simulink model "untitled1"  (R2025a)
settings: Solver=VariableStepAuto  StartTime=0.0  StopTime=36  MaxStep=1e-4  RelTol=1e-3
values from neighbouring files (symbols this model uses):
  alpha = 50    [Planning_Adaptive_LTV.m]
  beta = 5    [Planning_Adaptive_LTV.m]
  gamma = 10    [Planning_Adaptive_LTV.m]
  initial_positions_rad = rawJointPositions(1, :)'    [manipulator_sim.m]
  N = numel(theta_points_rad)    [create_LPV_linearizer.m]
  waypoints = pathObj.States(:, 1:2)    [Planning_Adaptive_LTV.m]
  x0 = zeros(10, 1)    [Planning_Adaptive_LTV.m]
undefined symbols (not defined in the file or in its folder): p, X, Y, Z
libraries: sm_lib x181, nesl_utility x29, fl_lib x3, simulink x2, eeGeneralControl x1
(part 1 of 5)
settings Model: Creator=chiar_zjcy1by  LastModifiedBy=chiar_zjcy1by

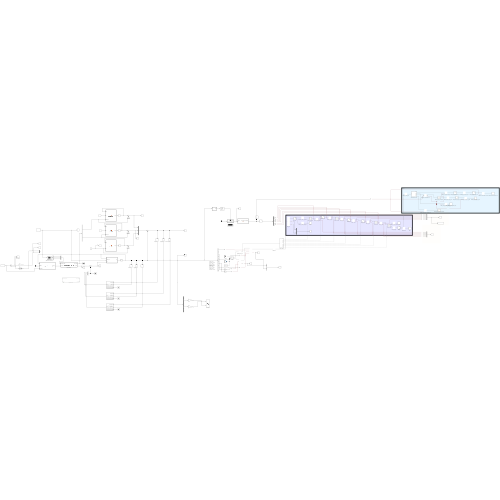
[thumbnail: Simulink's stored preview of the top-level diagram]
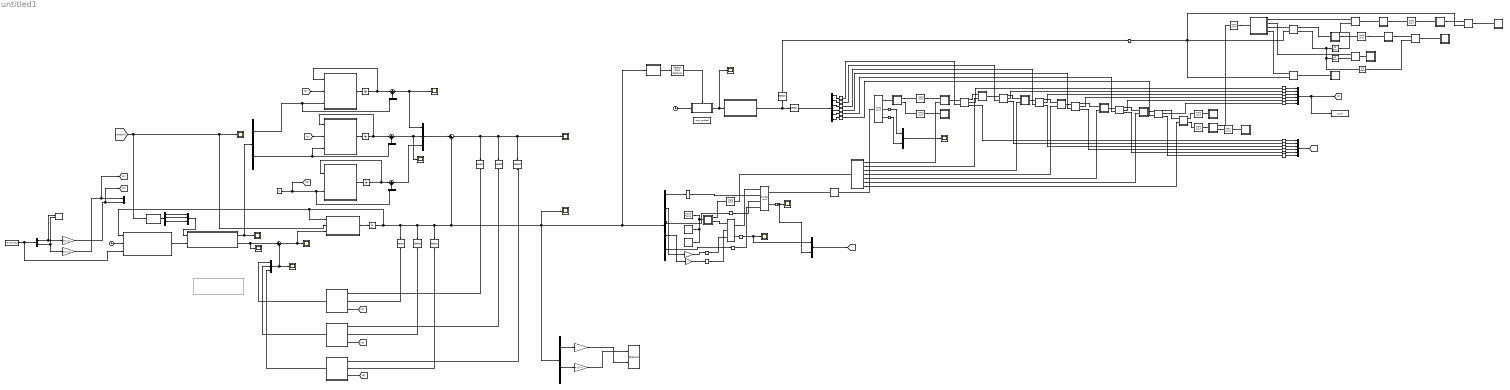
== system untitled1 ==
  note: MASTER JOINT
  note: Robotic Arm
  note: theta_x = x(1);
      | dot_theta_x = x(2);
      | phi_x = x(3);
      | dot_phi_x = x(4);
      | theta_y = x(5);
      | dot_theta_y = x(6);
      | phi_y = x(7);
      | dot_phi_y = x(8);
      | theta_z = x(9);
      | dot_theta_z = x(10);
  note: Gripper
  Cartesian Joint : sm_lib/Joints/Cartesian Joint  JointMode=Normal  CompositeWrenchDir=FollowerOnBase  CompositeWrenchFrame=BaseFrame  SenseConstraintForce=off  SenseConstraintTorque=off  SenseTotalForce=on  SenseTotalTorque=off  PxPositionTargetSpecify=off  PxPositionTargetPriority=High  PxPositionTargetValue=0  PxPositionTargetValueUnits=m  PxVelocityTargetSpecify=off  PxVelocityTargetPriority=High  PxVelocityTargetValue=0  PxVelocityTargetValueUnits=m/s  PxEquilibriumPosition=0  PxEquilibriumPositionUnits=m  PxSpringStiffness=0  PxSpringStiffnessUnits=N/m  PxDampingCoefficient=0  PxDampingCoefficientUnits=N/(m/s)  PxLowerLimitSpecify=off  PxLowerLimitBound=-1  PxLowerLimitBoundUnits=m  PxLowerLimitStiffness=1e6  PxLowerLimitStiffnessUnits=N/m  PxLowerLimitDamping=1e3  PxLowerLimitDampingUnits=N/(m/s)  PxLowerLimitTransitionRegionWidth=1e-4  PxLowerLimitTransitionRegionWidthUnits=m  PxUpperLimitSpecify=off  PxUpperLimitBound=1  PxUpperLimitBoundUnits=m  PxUpperLimitStiffness=1e6  PxUpperLimitStiffnessUnits=N/m  PxUpperLimitDamping=1e3  PxUpperLimitDampingUnits=N/(m/s)  PxUpperLimitTransitionRegionWidth=1e-4  PxUpperLimitTransitionRegionWidthUnits=m  PxTorqueActuationMode=ComputedTorque  PxMotionActuationMode=InputMotion  PxSensePosition=off  PxSenseVelocity=off  PxSenseAcceleration=off  PxSenseTorqueForce=off  PxSenseLowerLimitTorqueForce=off  PxSenseUpperLimitTorqueForce=off  PyPositionTargetSpecify=off  PyPositionTargetPriority=High  PyPositionTargetValue=0  PyPositionTargetValueUnits=m  PyVelocityTargetSpecify=off  PyVelocityTargetPriority=High  PyVelocityTargetValue=0  PyVelocityTargetValueUnits=m/s  PyEquilibriumPosition=0  PyEquilibriumPositionUnits=m  PySpringStiffness=0  PySpringStiffnessUnits=N/m  PyDampingCoefficient=0  PyDampingCoefficientUnits=N/(m/s)  PyLowerLimitSpecify=off  PyLowerLimitBound=-1  PyLowerLimitBoundUnits=m  PyLowerLimitStiffness=1e6  PyLowerLimitStiffnessUnits=N/m  PyLowerLimitDamping=1e3  PyLowerLimitDampingUnits=N/(m/s)  PyLowerLimitTransitionRegionWidth=1e-4  PyLowerLimitTransitionRegionWidthUnits=m  PyUpperLimitSpecify=off  PyUpperLimitBound=1  PyUpperLimitBoundUnits=m  PyUpperLimitStiffness=1e6  PyUpperLimitStiffnessUnits=N/m  PyUpperLimitDamping=1e3  PyUpperLimitDampingUnits=N/(m/s)  PyUpperLimitTransitionRegionWidth=1e-4  PyUpperLimitTransitionRegionWidthUnits=m  PyTorqueActuationMode=ComputedTorque  PyMotionActuationMode=InputMotion  PySensePosition=off  PySenseVelocity=off  PySenseAcceleration=off  PySenseTorqueForce=off  PySenseLowerLimitTorqueForce=off  PySenseUpperLimitTorqueForce=off  PzPositionTargetSpecify=off  PzPositionTargetPriority=High  PzPositionTargetValue=0  PzPositionTargetValueUnits=m  PzVelocityTargetSpecify=off  PzVelocityTargetPriority=High  PzVelocityTargetValue=0  PzVelocityTargetValueUnits=m/s  PzEquilibriumPosition=0  PzEquilibriumPositionUnits=m  PzSpringStiffness=0  PzSpringStiffnessUnits=N/m  PzDampingCoefficient=0  PzDampingCoefficientUnits=N/(m/s)  PzLowerLimitSpecify=off  PzLowerLimitBound=-1  PzLowerLimitBoundUnits=m  PzLowerLimitStiffness=1e6  PzLowerLimitStiffnessUnits=N/m  PzLowerLimitDamping=1e3  PzLowerLimitDampingUnits=N/(m/s)  PzLowerLimitTransitionRegionWidth=1e-4  PzLowerLimitTransitionRegionWidthUnits=m  PzUpperLimitSpecify=off  PzUpperLimitBound=1  PzUpperLimitBoundUnits=m  PzUpperLimitStiffness=1e6  PzUpperLimitStiffnessUnits=N/m  PzUpperLimitDamping=1e3  PzUpperLimitDampingUnits=N/(m/s)  PzUpperLimitTransitionRegionWidth=1e-4  PzUpperLimitTransitionRegionWidthUnits=m  PzTorqueActuationMode=NoTorque  PzMotionActuationMode=ComputedMotion  PzSensePosition=off  PzSenseVelocity=off  PzSenseAcceleration=off  PzSenseTorqueForce=off  PzSenseLowerLimitTorqueForce=off  PzSenseUpperLimitTorqueForce=off
  Clock : Clock
  Clock2 : Clock
  Constant1 : Constant  Value=0
  Data Store Memory1 : DataStoreMemory  DataStoreName=play_enbled  WriteAfterWriteMsg=warning  ShowAdditionalParam=off
  Demux : Demux  Outputs=2
  Demux1 : Demux  Outputs=2
  Demux2 : Demux  Outputs=10
  Demux3 : Demux  Outputs=6
  Demux4 : Demux  Outputs=10
  Demux5 : Demux  Outputs=6
  Detect Rise Positive : simulink/Logic and Bit Operations/Detect Rise Positive  vinit=0  OutDataTypeStr=boolean
  EQ generator1 : MATLAB Function  TreatAsAtomicUnit=on
  EQ generator3 : MATLAB Function  Commented=on  TreatAsAtomicUnit=on
  From Workspace3 : FromWorkspace  VariableName=waypoints_ts  SampleTime=0.01  OutputAfterFinalValue=Holding final value
  Gain : Gain  Gain=1/p.r_S
  Gain1 : Gain  Gain=-1/p.r_S
  Gain4 : Gain  Gain=p.r_S  Multiplication=Matrix(K*u)
  Gain5 : Gain  Gain=-p.r_S  Multiplication=Matrix(K*u)
  Gimbal Joint : sm_lib/Joints/Gimbal Joint  JointMode=Normal  CompositeWrenchDir=FollowerOnBase  CompositeWrenchFrame=BaseFrame  SenseConstraintForce=off  SenseConstraintTorque=off  SenseTotalForce=off  SenseTotalTorque=on  RxPositionTargetSpecify=off  RxPositionTargetPriority=High  RxPositionTargetValue=0  RxPositionTargetValueUnits=deg  RxVelocityTargetSpecify=off  RxVelocityTargetPriority=High  RxVelocityTargetValue=0  RxVelocityTargetValueUnits=deg/s  RxEquilibriumPosition=0  RxEquilibriumPositionUnits=deg  RxSpringStiffness=0  RxSpringStiffnessUnits=N*m/deg  RxDampingCoefficient=0  RxDampingCoefficientUnits=N*m/(deg/s)  RxLowerLimitSpecify=off  RxLowerLimitBound=-90  RxLowerLimitBoundUnits=deg  RxLowerLimitStiffness=1e4  RxLowerLimitStiffnessUnits=N*m/deg  RxLowerLimitDamping=10  RxLowerLimitDampingUnits=N*m/(deg/s)  RxLowerLimitTransitionRegionWidth=0.1  RxLowerLimitTransitionRegionWidthUnits=deg  RxUpperLimitSpecify=off  RxUpperLimitBound=90  RxUpperLimitBoundUnits=deg  RxUpperLimitStiffness=1e4  RxUpperLimitStiffnessUnits=N*m/deg  RxUpperLimitDamping=10  RxUpperLimitDampingUnits=N*m/(deg/s)  RxUpperLimitTransitionRegionWidth=0.1  RxUpperLimitTransitionRegionWidthUnits=deg  RxTorqueActuationMode=ComputedTorque  RxMotionActuationMode=InputMotion  RxSensePosition=off  RxSenseVelocity=off  RxSenseAcceleration=off  RxSenseTorqueForce=off  RxSenseLowerLimitTorqueForce=off  RxSenseUpperLimitTorqueForce=off  RyPositionTargetSpecify=off  RyPositionTargetPriority=High  RyPositionTargetValue=0  RyPositionTargetValueUnits=deg  RyVelocityTargetSpecify=off  RyVelocityTargetPriority=High  RyVelocityTargetValue=0  RyVelocityTargetValueUnits=deg/s  RyEquilibriumPosition=0  RyEquilibriumPositionUnits=deg  RySpringStiffness=0  RySpringStiffnessUnits=N*m/deg  RyDampingCoefficient=0  RyDampingCoefficientUnits=N*m/(deg/s)  RyLowerLimitSpecify=off  RyLowerLimitBound=-90  RyLowerLimitBoundUnits=deg  RyLowerLimitStiffness=1e4  RyLowerLimitStiffnessUnits=N*m/deg  RyLowerLimitDamping=10  RyLowerLimitDampingUnits=N*m/(deg/s)  RyLowerLimitTransitionRegionWidth=0.1  RyLowerLimitTransitionRegionWidthUnits=deg  RyUpperLimitSpecify=off  RyUpperLimitBound=90  RyUpperLimitBoundUnits=deg  RyUpperLimitStiffness=1e4  RyUpperLimitStiffnessUnits=N*m/deg  RyUpperLimitDamping=10  RyUpperLimitDampingUnits=N*m/(deg/s)  RyUpperLimitTransitionRegionWidth=0.1  RyUpperLimitTransitionRegionWidthUnits=deg  RyTorqueActuationMode=ComputedTorque  RyMotionActuationMode=InputMotion  RySensePosition=off  RySenseVelocity=off  RySenseAcceleration=off  RySenseTorqueForce=off  RySenseLowerLimitTorqueForce=off  RySenseUpperLimitTorqueForce=off  RzPositionTargetSpecify=off  RzPositionTargetPriority=High  RzPositionTargetValue=x0(1)  RzPositionTargetValueUnits=rad  RzVelocityTargetSpecify=off  RzVelocityTargetPriority=High  RzVelocityTargetValue=0  RzVelocityTargetValueUnits=deg/s  RzEquilibriumPosition=0  RzEquilibriumPositionUnits=deg  RzSpringStiffness=0  RzSpringStiffnessUnits=N*m/deg  RzDampingCoefficient=0  RzDampingCoefficientUnits=N*m/(deg/s)  RzLowerLimitSpecify=off  RzLowerLimitBound=-90  RzLowerLimitBoundUnits=deg  RzLowerLimitStiffness=1e4  RzLowerLimitStiffnessUnits=N*m/deg  RzLowerLimitDamping=10  RzLowerLimitDampingUnits=N*m/(deg/s)  RzLowerLimitTransitionRegionWidth=0.1  RzLowerLimitTransitionRegionWidthUnits=deg  RzUpperLimitSpecify=off  RzUpperLimitBound=90  RzUpperLimitBoundUnits=deg  RzUpperLimitStiffness=1e4  RzUpperLimitStiffnessUnits=N*m/deg  RzUpperLimitDamping=10  RzUpperLimitDampingUnits=N*m/(deg/s)  RzUpperLimitTransitionRegionWidth=0.1  RzUpperLimitTransitionRegionWidthUnits=deg  RzTorqueActuationMode=ComputedTorque  RzMotionActuationMode=InputMotion  RzSensePosition=off  RzSenseVelocity=off  RzSenseAcceleration=off  RzSenseTorqueForce=off  RzSenseLowerLimitTorqueForce=off  RzSenseUpperLimitTorqueForce=off
  Integrator : Integrator  InitialCondition=[0;0;0;0]-x0(1:4)
  Integrator2 : Integrator  InitialCondition=[0;0;0;0]-x0(5:8)
  Integrator3 : Integrator  InitialCondition=x0(9:10)
  Integrator4 : Integrator  InitialCondition=x0
  Low-Pass Filter (Discrete or Continuous) : eeGeneralControl/Low-Pass Filter (Discrete or Continuous)  K=1  T=0.03  B=inf  A=-inf  init_option=Inherited from block input  x0=0  Ts=-1
  MATLAB Function : MATLAB Function  TreatAsAtomicUnit=on
  MATLAB Function1 : MATLAB Function  TreatAsAtomicUnit=on
  MATLAB Function2 : MATLAB Function  TreatAsAtomicUnit=on
  MATLAB Function3 : MATLAB Function  TreatAsAtomicUnit=on
  MATLAB Function4 : MATLAB Function  TreatAsAtomicUnit=on
  MATLAB Function5 : MATLAB Function  TreatAsAtomicUnit=on
  MATLAB Function7 : MATLAB Function  TreatAsAtomicUnit=on
  MechanismConfiguration : sm_lib/Utilities/Mechanism Configuration  UniformGravity=Constant  GravityVector=[0, 0, -9]  GravityVectorUnits=m/s^2  LinearizationDelta=0.001  JointModeTransitionNonlinearIterations=2
  Multiply : Gain  Gain=p.r_S
  Multiply1 : Gain  Gain=-p.r_S
  Mux{,5,8..9} (4 alike) : Mux  Inputs=2
  Mux1 : Mux  Inputs=3
  Mux10 : Mux  Inputs=6
  Mux2 : Mux  Inputs=3
  Mux3 : Mux
  Mux4 : Mux
  Mux6 : Mux  Inputs=6
  Mux7 : Mux  Inputs=6
  PS Gain : fl_lib/Physical Signals/Functions/PS Gain  gain=-1
  PS Gain1 : fl_lib/Physical Signals/Functions/PS Gain  gain=-1
  PS Gain2 : fl_lib/Physical Signals/Functions/PS Gain  gain=-1
  PS-Simulink Converter{,1..15} (16 alike) : nesl_utility/PS-Simulink Converter  PhysicalDomain=network_engine_domain  SubClassName=ps_output  LeftPortType=input  RightPortType=output  PseudoPeriodic=off  Frequencies=[]  VectorFormat=inherit  Unit=inherit  AffineConversion=off
  Scope{,1..9,11,13,15} (13 alike) : Scope
      Scope settings: ActiveDisplayYMinimum=-44.711357738519766  ActiveDisplayYMaximum=6.09165695104528  DataLoggingVariableName=ScopeData18  DataLoggingSaveFormat=Array
      Scope1 settings: ActiveDisplayYMinimum=-1.6776166533839281  ActiveDisplayYMaximum=4.8671835129178067  DataLoggingSaveFormat=Array
      Scope11 settings: ActiveDisplayYMinimum=-5.0574559454104868  ActiveDisplayYMaximum=39.374571185756373  DataLoggingVariableName=ScopeData19  DataLoggingSaveFormat=Array
      Scope13 settings: ActiveDisplayYMinimum=-9.5230896865540743E+6  ActiveDisplayYMaximum=3.9326641649716813E+6  DataLoggingVariableName=ScopeData22  DataLoggingSaveFormat=Array
      Scope15 settings: ActiveDisplayYMinimum=-1  ActiveDisplayYMaximum=1  DataLoggingVariableName=ScopeData24  DataLoggingSaveFormat=Array
      Scope2 settings: ActiveDisplayYMinimum=-27.920029110961494  ActiveDisplayYMaximum=123.73506241979986  DataLoggingSaveFormat=Array
      Scope3 settings: ActiveDisplayYMinimum=-129.69624805004366  ActiveDisplayYMaximum=65.56202970679449  DataLoggingVariableName=ScopeData3  DataLoggingSaveFormat=Array
      Scope4 settings: ActiveDisplayYMinimum=4.7249999999643411  ActiveDisplayYMaximum=6.7249999999643411  DataLoggingVariableName=ScopeData4  DataLoggingSaveFormat=Array
      Scope5 settings: ActiveDisplayYMinimum=-469.4220082836041  ActiveDisplayYMaximum=537.72627814043176  DataLoggingVariableName=ScopeData5  DataLoggingSaveFormat=Array
      Scope6 settings: ActiveDisplayYMinimum=-2.6775524020195045E-9  ActiveDisplayYMaximum=2.4097971618175507E-8  DataLoggingVariableName=ScopeData9
      Scope7 settings: ActiveDisplayYMinimum=-1.1832122709621713E+6  ActiveDisplayYMaximum=131468.03013649114  DataLoggingVariableName=ScopeData21
      Scope8 settings: ActiveDisplayYMinimum=-235.53516320104924  ActiveDisplayYMaximum=579.96367387225951  DataLoggingVariableName=ScopeData10  DataLoggingSaveFormat=Array
      Scope9 settings: ActiveDisplayYMinimum=-2.4063172942734425  ActiveDisplayYMaximum=0.9316742644861904  DataLoggingVariableName=ScopeData11  DataLoggingSaveFormat=Array
  Selector1 : Selector  InputPortWidth=10  IndexOptions=Index vector (dialog)  Indices=[9 10]  OutputSizes=1
  Selector10 : Selector  InputPortWidth=7  IndexOptions=Index vector (dialog)  Indices=[4]  OutputSizes=1
  Selector11 : Selector  InputPortWidth=7  IndexOptions=Index vector (dialog)  Indices=[1 2 3 5 6 7]  OutputSizes=1
  Selector2 : Selector  InputPortWidth=10  IndexOptions=Index vector (dialog)  Indices=[5 6 7 8]  OutputSizes=1
  Selector3 : Selector  InputPortWidth=10  IndexOptions=Index vector (dialog)  Indices=[1 2 3 4]  OutputSizes=1
  Selector4 : Selector  InputPortWidth=10  IndexOptions=Index vector (dialog)  Indices=[9 10]  OutputSizes=1
  Selector5 : Selector  InputPortWidth=10  IndexOptions=Index vector (dialog)  Indices=[5 6 7 8]  OutputSizes=1
  Selector9 : Selector  InputPortWidth=10  IndexOptions=Index vector (dialog)  Indices=[1 2 3 4]  OutputSizes=1
  Simulink-PS Converter{,1..8,11,13} (11 alike) : nesl_utility/Simulink-PS Converter  PhysicalDomain=network_engine_domain  SubClassName=ps_input  LeftPortType=input  RightPortType=output  PseudoPeriodic=off  Frequencies=[]  NoiseDistribution=none  NoiseParameters=[]  Unit=1  AffineConversion=off  FilteringAndDerivatives=filter  SimscapeFilterOrder=2  InputFilterTimeConstant=0.001  UdotUserProvided=0
  Simulink-PS Converter10 : nesl_utility/Simulink-PS Converter  PhysicalDomain=network_engine_domain  SubClassName=ps_input  LeftPortType=input  RightPortType=output  PseudoPeriodic=off  Frequencies=[]  NoiseDistribution=none  NoiseParameters=[]  Unit=1  AffineConversion=off  FilteringAndDerivatives=filter  SimscapeFilterOrder=2  InputFilterTimeConstant=0.001  UdotUserProvided=2
  Solver Configuration : nesl_utility/Solver Configuration  PhysicalDomain=network_engine_domain  SubClassName=solver  LeftPortType=input  RightPortType=generic  Tones=[]  Harmonics=[]  SimulateNoise=off  Profile=off  UseLocalSampling=off  EnableSwitchedLinearOptims=on  FrequencyDomain=off  UseCCode=off  RelTol=0.001  AbsTol=0.001  MinStep=1e-09  ToWorkspace=off  RevertToSquareIcSolve=off  NumHomotopyIterations=100  PhasorMode=off  PhasorModeNumHarmonics=1  ConsistencySolver=NEWTON_XTOL_AFTER_FTOL  IndexReductionMethod=DerivativeReplacement  DoDC=off  ResidualTolerance=1e-09  ConsistencyTolSource=GLOBAL  ConsistencyAbsTol=0.001  ConsistencyRelTol=0.001  ConsistencyTolFactor=0.001  UseLocalSolver=off  LocalSolverChoice=NE_BACKWARD_EULER_ADVANCER  ResolveIndetEquations=on  FunctionEvalNumThread=1  LocalSolverSampleTime=0.001  DoFixedCost=off  MaxNonlinIter=3  MaxModeIter=2  ComputeImpulses=off  ImpulseIterations=2  LinearAlgebra=auto  LinearAlgebraNumThread=0  EquationFormulation=NE_TIME_EF  DelaysMemoryBudget=1024  AutomaticFiltering=on  FilteringTimeConstant=0.01  PartitionStorageMethod=AS_NEEDED  PartitionMemoryBudget=1024  PartitionMethod=ROBUST  MultibodyUseLocalSolver=off  MultibodyLocalSolverChoice=ODE1  MultibodyLocalSolverSampleTime=0.001
  Subsystem : Subsystem
  Subsystem1 : Subsystem
  Subsystem2 : Subsystem
  Sum{,2..4} (4 alike) : Sum  Inputs=|++
  Sum1 : Sum  Inputs=|+-
  To Workspace : ToWorkspace  VariableName=q_sim  SaveFormat=Structure With Time  SampleTime=-1
  Transform : sm_lib/Frames and Transforms/Rigid Transform  RotationMethod=RotationSequence  FollAlignAxisA=+X  BaseAlignAxisA=+Y  FollAlignAxisB=+Y  BaseAlignAxisB=+Z  RotationStandardAxis=+Z  RotationAngle=0  RotationAngleUnits=deg  RotationArbitraryAxis=[0 0 1]  RotationSequenceAxes=BaseAxes  RotationSequence=XYZ  RotationSequenceAngles=[0, 0, 0]  RotationSequenceAnglesUnits=rad  RotationMatrix=[1 0 0;0 1 0;0 0 1]  Quaternion=[1 0 0 0]  TranslationMethod=Cartesian  TranslationCartesianOffset=[0, 0, 0.05]  TranslationCartesianOffsetUnits=m  TranslationStandardAxis=+Z  TranslationStandardOffset=0  TranslationStandardOffsetUnits=m  TranslationROffset=0  TranslationROffsetUnits=m  TranslationThetaOffset=0  TranslationThetaOffsetUnits=deg  TranslationZOffset=0  TranslationZOffsetUnits=m
  Triggered Subsystem : Subsystem  TreatAsAtomicUnit=on
  World : sm_lib/Frames and Transforms/World Frame
  XY Graph : Record  NumPorts=2.0  FileSettingsInternal="{\"entries\":[{\"content\":{\"excelSettings\":{\"content\":{},\"type\":\"Streamout.ExcelSettings\"},\"parquetSettings\":{\"content\":{},\"type\":\"Streamout.ParquetSettings\"}},\"type\":\"Streamout.FileSettingStorage\",\"uuid\":\"\"}],\"packageUris\":[\"http:\\/\\/schema.mathworks.com\\/mf0\\/streamout_blocks\\/R2020a\"],\"version\":\"1.0\"}"  FrameSettings=[0, 0]  Layout=[1 1]  SignalsInternal="{\"entries\":[{\"content\":{\"signals\":[{\"content\":{\"blockPath\":[],\"dimensions\":[1,1],\"domain\":\"\",\"lineColor\":\"#a2142f\",\"plots\":[ 1 ],\"port\":1,\"sid\":[\"\"],\"signalID\":1,\"signalName\":\"r2\"},\"type\":\"RecordBlkView.Signal\",\"uuid\":\"\"},{\"content\":{\"blockPath\":[],\"dimensions\":[1,1],\"domain\":\"\",\"lineColor\":\"#139fff\",\"plots\":[ 1 ],\"port\":2,\"sid\":[\"\"],\"signalID\":2,\"signalName\":\"r2\"},\"type\":\"RecordBlkView.Signal\",\"uuid\":\"\"}]},\"type\":\"RecordBlkView.InputSignals\",\"uuid\":\"\"}],\"packageUris\":[\"http:\\/\\/schema.mathworks.com\\/mf0\\/streamout_blocks\\/R2020a\"],\"version\":\"1.0\"}"  VisualizationBindings="{\"xyplotplugin\":{\"info\":[{\"series\":[{\"bindingParametersList\":[{\"parameter\":\"X-Axis\",\"signalID\":1,\"signalName\":\"r2\"},{\"parameter\":\"Y-Axis\",\"signalID\":2,\"signalName\":\"r2\"}],\"seriesID\":0}],\"subplotID\":1}]}}"  CompatibilityTag=XY
  XY Graph1 : Record  NumPorts=2.0  FileSettingsInternal="{\"entries\":[{\"content\":{\"excelSettings\":{\"content\":{},\"type\":\"Streamout.ExcelSettings\"},\"parquetSettings\":{\"content\":{},\"type\":\"Streamout.ParquetSettings\"}},\"type\":\"Streamout.FileSettingStorage\",\"uuid\":\"\"}],\"packageUris\":[\"http:\\/\\/schema.mathworks.com\\/mf0\\/streamout_blocks\\/R2020a\"],\"version\":\"1.0\"}"  FrameSettings=[0, 0]  Layout=[1 1]  SignalsInternal="{\"entries\":[{\"content\":{\"signals\":[{\"content\":{\"blockPath\":[],\"dimensions\":[1],\"domain\":\"\",\"lineColor\":\"#a2142f\",\"plots\":[ 1 ],\"port\":1,\"sid\":[\"\"],\"signalID\":1,\"signalName\":\"Demux:1\"},\"type\":\"RecordBlkView.Signal\",\"uuid\":\"\"},{\"content\":{\"blockPath\":[],\"dimensions\":[1],\"domain\":\"\",\"lineColor\":\"#139fff\",\"plots\":[ 1 ],\"port\":2,\"sid\":[\"\"],\"signalID\":2,\"signalName\":\"Demux:2\"},\"type\":\"RecordBlkView.Signal\",\"uuid\":\"\"}]},\"type\":\"RecordBlkView.InputSignals\",\"uuid\":\"\"}],\"packageUris\":[\"http:\\/\\/schema.mathworks.com\\/mf0\\/streamout_blocks\\/R2020a\"],\"version\":\"1.0\"}"  VisualizationBindings="{\"xyplotplugin\":{\"info\":[{\"series\":[{\"bindingParametersList\":[{\"parameter\":\"X-Axis\",\"signalID\":1,\"signalName\":\"Demux:1\"},{\"parameter\":\"Y-Axis\",\"signalID\":2,\"signalName\":\"Demux:2\"}],\"seriesID\":0}],\"subplotID\":1}]}}"  CompatibilityTag=XY
  base : Subsystem
  base_joint : sm_lib/Joints/Weld Joint  JointMode=Normal  CompositeWrenchDir=FollowerOnBase  CompositeWrenchFrame=BaseFrame  SenseConstraintForce=off  SenseConstraintTorque=off  SenseTotalForce=on  SenseTotalTorque=on
  base_link : Subsystem
  base_link_base_fixed_joint : sm_lib/Joints/Weld Joint  JointMode=Normal  CompositeWrenchDir=FollowerOnBase  CompositeWrenchFrame=BaseFrame  SenseConstraintForce=off  SenseConstraintTorque=off  SenseTotalForce=off  SenseTotalTorque=off
  base_link_base_link_inertia : sm_lib/Joints/Weld Joint  JointMode=Normal  CompositeWrenchDir=FollowerOnBase  CompositeWrenchFrame=BaseFrame  SenseConstraintForce=off  SenseConstraintTorque=off  SenseTotalForce=off  SenseTotalTorque=off
  base_link_inertia : Subsystem
  elbow_joint : sm_lib/Joints/Revolute Joint  JointMode=Normal  CompositeWrenchDir=FollowerOnBase  CompositeWrenchFrame=BaseFrame  SenseConstraintForce=off  SenseConstraintTorque=off  SenseTotalForce=off  SenseTotalTorque=off  PositionTargetSpecify=on  PositionTargetPriority=High  PositionTargetValue=initial_positions_rad(3)  PositionTargetValueUnits=rad  VelocityTargetSpecify=off  VelocityTargetPriority=High  VelocityTargetValue=0  VelocityTargetValueUnits=deg/s  EquilibriumPosition=0  EquilibriumPositionUnits=deg  SpringStiffness=0  SpringStiffnessUnits=N*m/deg  DampingCoefficient=0  DampingCoefficientUnits=kg*m^2/(rad*s)  LowerLimitSpecify=off  LowerLimitBound=-3.141592653589793  LowerLimitBoundUnits=rad  LowerLimitStiffness=1e4  LowerLimitStiffnessUnits=N*m/deg  LowerLimitDamping=10  LowerLimitDampingUnits=N*m/(deg/s)  LowerLimitTransitionRegionWidth=0.1  LowerLimitTransitionRegionWidthUnits=deg  UpperLimitSpecify=off  UpperLimitBound=3.141592653589793  UpperLimitBoundUnits=rad  UpperLimitStiffness=1e4  UpperLimitStiffnessUnits=N*m/deg  UpperLimitDamping=10  UpperLimitDampingUnits=N*m/(deg/s)  UpperLimitTransitionRegionWidth=0.1  UpperLimitTransitionRegionWidthUnits=deg  TorqueActuationMode=ComputedTorque  MotionActuationMode=InputMotion  SensePosition=on  SenseVelocity=on  SenseAcceleration=off  SenseTorqueForce=off  SenseLowerLimitTorqueForce=off  SenseUpperLimitTorqueForce=off
  flange : Subsystem
  flange_tool0 : sm_lib/Joints/Weld Joint  JointMode=Normal  CompositeWrenchDir=FollowerOnBase  CompositeWrenchFrame=BaseFrame  SenseConstraintForce=off  SenseConstraintTorque=off  SenseTotalForce=off  SenseTotalTorque=off
  forearm_link : Subsystem
  ft_frame : Subsystem
  ground_plane : Subsystem
  ground_plane_joint : sm_lib/Joints/Weld Joint  JointMode=Normal  CompositeWrenchDir=FollowerOnBase  CompositeWrenchFrame=BaseFrame  SenseConstraintForce=off  SenseConstraintTorque=off  SenseTotalForce=off  SenseTotalTorque=off
  robotiq_85_base_joint : sm_lib/Joints/Weld Joint  JointMode=Normal  CompositeWrenchDir=FollowerOnBase  CompositeWrenchFrame=BaseFrame  SenseConstraintForce=off  SenseConstraintTorque=off  SenseTotalForce=off  SenseTotalTorque=off
  robotiq_85_base_link : Subsystem
  robotiq_85_left_finger_joint : sm_lib/Joints/Weld Joint  JointMode=Normal  CompositeWrenchDir=FollowerOnBase  CompositeWrenchFrame=BaseFrame  SenseConstraintForce=off  SenseConstraintTorque=off  SenseTotalForce=off  SenseTotalTorque=off
  robotiq_85_left_finger_link : Subsystem
  robotiq_85_left_finger_tip_joint : sm_lib/Joints/Revolute Joint  JointMode=Normal  CompositeWrenchDir=FollowerOnBase  CompositeWrenchFrame=BaseFrame  SenseConstraintForce=off  SenseConstraintTorque=off  SenseTotalForce=off  SenseTotalTorque=off  PositionTargetSpecify=on  PositionTargetPriority=High  PositionTargetValue=0  PositionTargetValueUnits=rad  VelocityTargetSpecify=off  VelocityTargetPriority=High  VelocityTargetValue=0  VelocityTargetValueUnits=deg/s  EquilibriumPosition=0  EquilibriumPositionUnits=deg  SpringStiffness=0  SpringStiffnessUnits=N*m/deg  DampingCoefficient=0  DampingCoefficientUnits=kg*m^2/(rad*s)  LowerLimitSpecify=off  LowerLimitBound=-90  LowerLimitBoundUnits=deg  LowerLimitStiffness=1e4  LowerLimitStiffnessUnits=N*m/deg  LowerLimitDamping=10  LowerLimitDampingUnits=N*m/(deg/s)  LowerLimitTransitionRegionWidth=0.1  LowerLimitTransitionRegionWidthUnits=deg  UpperLimitSpecify=off  UpperLimitBound=90  UpperLimitBoundUnits=deg  UpperLimitStiffness=1e4  UpperLimitStiffnessUnits=N*m/deg  UpperLimitDamping=10  UpperLimitDampingUnits=N*m/(deg/s)  UpperLimitTransitionRegionWidth=0.1  UpperLimitTransitionRegionWidthUnits=deg  TorqueActuationMode=ComputedTorque  MotionActuationMode=InputMotion  SensePosition=off  SenseVelocity=off  SenseAcceleration=off  SenseTorqueForce=off  SenseLowerLimitTorqueForce=off  SenseUpperLimitTorqueForce=off
  robotiq_85_left_finger_tip_link : Subsystem
  robotiq_85_left_inner_knuckle_joint : sm_lib/Joints/Revolute Joint  JointMode=Normal  CompositeWrenchDir=FollowerOnBase  CompositeWrenchFrame=BaseFrame  SenseConstraintForce=off  SenseConstraintTorque=off  SenseTotalForce=off  SenseTotalTorque=off  PositionTargetSpecify=off  PositionTargetPriority=High  PositionTargetValue=0  PositionTargetValueUnits=rad  VelocityTargetSpecify=off  VelocityTargetPriority=High  VelocityTargetValue=0  VelocityTargetValueUnits=deg/s  EquilibriumPosition=0  EquilibriumPositionUnits=deg  SpringStiffness=0  SpringStiffnessUnits=N*m/deg  DampingCoefficient=0  DampingCoefficientUnits=kg*m^2/(rad*s)  LowerLimitSpecify=off  LowerLimitBound=-90  LowerLimitBoundUnits=deg  LowerLimitStiffness=1e4  LowerLimitStiffnessUnits=N*m/deg  LowerLimitDamping=10  LowerLimitDampingUnits=N*m/(deg/s)  LowerLimitTransitionRegionWidth=0.1  LowerLimitTransitionRegionWidthUnits=deg  UpperLimitSpecify=off  UpperLimitBound=90  UpperLimitBoundUnits=deg  UpperLimitStiffness=1e4  UpperLimitStiffnessUnits=N*m/deg  UpperLimitDamping=10  UpperLimitDampingUnits=N*m/(deg/s)  UpperLimitTransitionRegionWidth=0.1  UpperLimitTransitionRegionWidthUnits=deg  TorqueActuationMode=ComputedTorque  MotionActuationMode=InputMotion  SensePosition=off  SenseVelocity=off  SenseAcceleration=off  SenseTorqueForce=off  SenseLowerLimitTorqueForce=off  SenseUpperLimitTorqueForce=off
  robotiq_85_left_inner_knuckle_link : Subsystem
  robotiq_85_left_knuckle_joint : sm_lib/Joints/Revolute Joint  JointMode=Normal  CompositeWrenchDir=FollowerOnBase  CompositeWrenchFrame=BaseFrame  SenseConstraintForce=off  SenseConstraintTorque=off  SenseTotalForce=off  SenseTotalTorque=off  PositionTargetSpecify=on  PositionTargetPriority=High  PositionTargetValue=initial_positions_rad(4)  PositionTargetValueUnits=rad  VelocityTargetSpecify=off  VelocityTargetPriority=High  VelocityTargetValue=0  VelocityTargetValueUnits=deg/s  EquilibriumPosition=0  EquilibriumPositionUnits=deg  SpringStiffness=0  SpringStiffnessUnits=N*m/deg  DampingCoefficient=0  DampingCoefficientUnits=kg*m^2/(rad*s)  LowerLimitSpecify=on  LowerLimitBound=0  LowerLimitBoundUnits=rad  LowerLimitStiffness=1e4  LowerLimitStiffnessUnits=N*m/deg  LowerLimitDamping=10  LowerLimitDampingUnits=N*m/(deg/s)  LowerLimitTransitionRegionWidth=0.1  LowerLimitTransitionRegionWidthUnits=deg  UpperLimitSpecify=on  UpperLimitBound=0.8  UpperLimitBoundUnits=rad  UpperLimitStiffness=1e4  UpperLimitStiffnessUnits=N*m/deg  UpperLimitDamping=10  UpperLimitDampingUnits=N*m/(deg/s)  UpperLimitTransitionRegionWidth=0.1  UpperLimitTransitionRegionWidthUnits=deg  TorqueActuationMode=ComputedTorque  MotionActuationMode=InputMotion  SensePosition=on  SenseVelocity=off  SenseAcceleration=off  SenseTorqueForce=off  SenseLowerLimitTorqueForce=off  SenseUpperLimitTorqueForce=off
  robotiq_85_left_knuckle_link : Subsystem
  robotiq_85_right_finger_joint : sm_lib/Joints/Weld Joint  JointMode=Normal  CompositeWrenchDir=FollowerOnBase  CompositeWrenchFrame=BaseFrame  SenseConstraintForce=off  SenseConstraintTorque=off  SenseTotalForce=off  SenseTotalTorque=off
  robotiq_85_right_finger_link : Subsystem
  robotiq_85_right_finger_tip_joint : sm_lib/Joints/Revolute Joint  JointMode=Normal  CompositeWrenchDir=FollowerOnBase  CompositeWrenchFrame=BaseFrame  SenseConstraintForce=off  SenseConstraintTorque=off  SenseTotalForce=off  SenseTotalTorque=off  PositionTargetSpecify=on  PositionTargetPriority=High  PositionTargetValue=0  PositionTargetValueUnits=rad  VelocityTargetSpecify=off  VelocityTargetPriority=High  VelocityTargetValue=0  VelocityTargetValueUnits=deg/s  EquilibriumPosition=0  EquilibriumPositionUnits=deg  SpringStiffness=0  SpringStiffnessUnits=N*m/deg  DampingCoefficient=0  DampingCoefficientUnits=kg*m^2/(rad*s)  LowerLimitSpecify=off  LowerLimitBound=-90  LowerLimitBoundUnits=deg  LowerLimitStiffness=1e4  LowerLimitStiffnessUnits=N*m/deg  LowerLimitDamping=10  LowerLimitDampingUnits=N*m/(deg/s)  LowerLimitTransitionRegionWidth=0.1  LowerLimitTransitionRegionWidthUnits=deg  UpperLimitSpecify=off  UpperLimitBound=90  UpperLimitBoundUnits=deg  UpperLimitStiffness=1e4  UpperLimitStiffnessUnits=N*m/deg  UpperLimitDamping=10  UpperLimitDampingUnits=N*m/(deg/s)  UpperLimitTransitionRegionWidth=0.1  UpperLimitTransitionRegionWidthUnits=deg  TorqueActuationMode=ComputedTorque  MotionActuationMode=InputMotion  SensePosition=off  SenseVelocity=off  SenseAcceleration=off  SenseTorqueForce=off  SenseLowerLimitTorqueForce=off  SenseUpperLimitTorqueForce=off
  robotiq_85_right_finger_tip_link : Subsystem
  robotiq_85_right_inner_knuckle_joint : sm_lib/Joints/Revolute Joint  JointMode=Normal  CompositeWrenchDir=FollowerOnBase  CompositeWrenchFrame=BaseFrame  SenseConstraintForce=off  SenseConstraintTorque=off  SenseTotalForce=off  SenseTotalTorque=off  PositionTargetSpecify=off  PositionTargetPriority=High  PositionTargetValue=0  PositionTargetValueUnits=rad  VelocityTargetSpecify=off  VelocityTargetPriority=High  VelocityTargetValue=0  VelocityTargetValueUnits=deg/s  EquilibriumPosition=0  EquilibriumPositionUnits=deg  SpringStiffness=0  SpringStiffnessUnits=N*m/deg  DampingCoefficient=0  DampingCoefficientUnits=kg*m^2/(rad*s)  LowerLimitSpecify=off  LowerLimitBound=-90  LowerLimitBoundUnits=deg  LowerLimitStiffness=1e4  LowerLimitStiffnessUnits=N*m/deg  LowerLimitDamping=10  LowerLimitDampingUnits=N*m/(deg/s)  LowerLimitTransitionRegionWidth=0.1  LowerLimitTransitionRegionWidthUnits=deg  UpperLimitSpecify=off  UpperLimitBound=90  UpperLimitBoundUnits=deg  UpperLimitStiffness=1e4  UpperLimitStiffnessUnits=N*m/deg  UpperLimitDamping=10  UpperLimitDampingUnits=N*m/(deg/s)  UpperLimitTransitionRegionWidth=0.1  UpperLimitTransitionRegionWidthUnits=deg  TorqueActuationMode=ComputedTorque  MotionActuationMode=InputMotion  SensePosition=off  SenseVelocity=off  SenseAcceleration=off  SenseTorqueForce=off  SenseLowerLimitTorqueForce=off  SenseUpperLimitTorqueForce=off
  robotiq_85_right_inner_knuckle_link : Subsystem
  robotiq_85_right_knuckle_joint : sm_lib/Joints/Revolute Joint  JointMode=Normal  CompositeWrenchDir=FollowerOnBase  CompositeWrenchFrame=BaseFrame  SenseConstraintForce=off  SenseConstraintTorque=off  SenseTotalForce=off  SenseTotalTorque=off  PositionTargetSpecify=off  PositionTargetPriority=High  PositionTargetValue=0  PositionTargetValueUnits=rad  VelocityTargetSpecify=off  VelocityTargetPriority=High  VelocityTargetValue=0  VelocityTargetValueUnits=deg/s  EquilibriumPosition=0  EquilibriumPositionUnits=deg  SpringStiffness=0  SpringStiffnessUnits=N*m/deg  DampingCoefficient=0  DampingCoefficientUnits=kg*m^2/(rad*s)  LowerLimitSpecify=on  LowerLimitBound=-0.8  LowerLimitBoundUnits=rad  LowerLimitStiffness=1e4  LowerLimitStiffnessUnits=N*m/deg  LowerLimitDamping=10  LowerLimitDampingUnits=N*m/(deg/s)  LowerLimitTransitionRegionWidth=0.1  LowerLimitTransitionRegionWidthUnits=deg  UpperLimitSpecify=on  UpperLimitBound=0  UpperLimitBoundUnits=rad  UpperLimitStiffness=1e4  UpperLimitStiffnessUnits=N*m/deg  UpperLimitDamping=10  UpperLimitDampingUnits=N*m/(deg/s)  UpperLimitTransitionRegionWidth=0.1  UpperLimitTransitionRegionWidthUnits=deg  TorqueActuationMode=ComputedTorque  MotionActuationMode=InputMotion  SensePosition=off  SenseVelocity=off  SenseAcceleration=off  SenseTorqueForce=off  SenseLowerLimitTorqueForce=off  SenseUpperLimitTorqueForce=off
  robotiq_85_right_knuckle_link : Subsystem
  shoulder_lift_joint : sm_lib/Joints/Revolute Joint  JointMode=Normal  CompositeWrenchDir=FollowerOnBase  CompositeWrenchFrame=BaseFrame  SenseConstraintForce=off  SenseConstraintTorque=off  SenseTotalForce=off  SenseTotalTorque=off  PositionTargetSpecify=on  PositionTargetPriority=High  PositionTargetValue=initial_positions_rad(2)  PositionTargetValueUnits=rad  VelocityTargetSpecify=off  VelocityTargetPriority=High  VelocityTargetValue=0  VelocityTargetValueUnits=deg/s  EquilibriumPosition=0  EquilibriumPositionUnits=deg  SpringStiffness=0  SpringStiffnessUnits=N*m/deg  DampingCoefficient=0  DampingCoefficientUnits=kg*m^2/(rad*s)  LowerLimitSpecify=on  LowerLimitBound=-6.283185307179586  LowerLimitBoundUnits=rad  LowerLimitStiffness=1e4  LowerLimitStiffnessUnits=N*m/deg  LowerLimitDamping=10  LowerLimitDampingUnits=N*m/(deg/s)  LowerLimitTransitionRegionWidth=0.1  LowerLimitTransitionRegionWidthUnits=deg  UpperLimitSpecify=on  UpperLimitBound=6.283185307179586  UpperLimitBoundUnits=rad  UpperLimitStiffness=1e4  UpperLimitStiffnessUnits=N*m/deg  UpperLimitDamping=10  UpperLimitDampingUnits=N*m/(deg/s)  UpperLimitTransitionRegionWidth=0.1  UpperLimitTransitionRegionWidthUnits=deg  TorqueActuationMode=ComputedTorque  MotionActuationMode=InputMotion  SensePosition=on  SenseVelocity=on  SenseAcceleration=off  SenseTorqueForce=off  SenseLowerLimitTorqueForce=off  SenseUpperLimitTorqueForce=off
  shoulder_link : Subsystem
  shoulder_pan_joint : sm_lib/Joints/Revolute Joint  JointMode=Normal  CompositeWrenchDir=FollowerOnBase  CompositeWrenchFrame=BaseFrame  SenseConstraintForce=off  SenseConstraintTorque=off  SenseTotalForce=off  SenseTotalTorque=off  PositionTargetSpecify=on  PositionTargetPriority=High  PositionTargetValue=initial_positions_rad(1)  PositionTargetValueUnits=rad  VelocityTargetSpecify=off  VelocityTargetPriority=High  VelocityTargetValue=0  VelocityTargetValueUnits=deg/s  EquilibriumPosition=0  EquilibriumPositionUnits=deg  SpringStiffness=0  SpringStiffnessUnits=N*m/deg  DampingCoefficient=0  DampingCoefficientUnits=kg*m^2/(rad*s)  LowerLimitSpecify=on  LowerLimitBound=-6.283185307179586  LowerLimitBoundUnits=rad  LowerLimitStiffness=1e4  LowerLimitStiffnessUnits=N*m/deg  LowerLimitDamping=10  LowerLimitDampingUnits=N*m/(deg/s)  LowerLimitTransitionRegionWidth=0.1  LowerLimitTransitionRegionWidthUnits=deg  UpperLimitSpecify=on  UpperLimitBound=6.283185307179586  UpperLimitBoundUnits=rad  UpperLimitStiffness=1e4  UpperLimitStiffnessUnits=N*m/deg  UpperLimitDamping=10  UpperLimitDampingUnits=N*m/(deg/s)  UpperLimitTransitionRegionWidth=0.1  UpperLimitTransitionRegionWidthUnits=deg  TorqueActuationMode=ComputedTorque  MotionActuationMode=InputMotion  SensePosition=on  SenseVelocity=on  SenseAcceleration=off  SenseTorqueForce=off  SenseLowerLimitTorqueForce=off  SenseUpperLimitTorqueForce=off
  tool0 : Subsystem
  upper_arm_link : Subsystem
  world : Subsystem
  wrist_1_joint : sm_lib/Joints/Revolute Joint  JointMode=Normal  CompositeWrenchDir=FollowerOnBase  CompositeWrenchFrame=BaseFrame  SenseConstraintForce=off  SenseConstraintTorque=off  SenseTotalForce=off  SenseTotalTorque=off  PositionTargetSpecify=on  PositionTargetPriority=High  PositionTargetValue=initial_positions_rad(5)  PositionTargetValueUnits=rad  VelocityTargetSpecify=off  VelocityTargetPriority=High  VelocityTargetValue=0  VelocityTargetValueUnits=deg/s  EquilibriumPosition=0  EquilibriumPositionUnits=deg  SpringStiffness=0  SpringStiffnessUnits=N*m/deg  DampingCoefficient=0  DampingCoefficientUnits=kg*m^2/(rad*s)  LowerLimitSpecify=on  LowerLimitBound=-6.283185307179586  LowerLimitBoundUnits=rad  LowerLimitStiffness=1e4  LowerLimitStiffnessUnits=N*m/deg  LowerLimitDamping=10  LowerLimitDampingUnits=N*m/(deg/s)  LowerLimitTransitionRegionWidth=0.1  LowerLimitTransitionRegionWidthUnits=deg  UpperLimitSpecify=on  UpperLimitBound=6.283185307179586  UpperLimitBoundUnits=rad  UpperLimitStiffness=1e4  UpperLimitStiffnessUnits=N*m/deg  UpperLimitDamping=10  UpperLimitDampingUnits=N*m/(deg/s)  UpperLimitTransitionRegionWidth=0.1  UpperLimitTransitionRegionWidthUnits=deg  TorqueActuationMode=ComputedTorque  MotionActuationMode=InputMotion  SensePosition=on  SenseVelocity=on  SenseAcceleration=off  SenseTorqueForce=off  SenseLowerLimitTorqueForce=off  SenseUpperLimitTorqueForce=off
  wrist_1_link : Subsystem
  wrist_2_joint : sm_lib/Joints/Revolute Joint  JointMode=Normal  CompositeWrenchDir=FollowerOnBase  CompositeWrenchFrame=BaseFrame  SenseConstraintForce=off  SenseConstraintTorque=off  SenseTotalForce=off  SenseTotalTorque=off  PositionTargetSpecify=on  PositionTargetPriority=High  PositionTargetValue=initial_positions_rad(6)  PositionTargetValueUnits=rad  VelocityTargetSpecify=off  VelocityTargetPriority=High  VelocityTargetValue=0  VelocityTargetValueUnits=deg/s  EquilibriumPosition=0  EquilibriumPositionUnits=deg  SpringStiffness=0  SpringStiffnessUnits=N*m/deg  DampingCoefficient=0  DampingCoefficientUnits=kg*m^2/(rad*s)  LowerLimitSpecify=on  LowerLimitBound=-6.283185307179586  LowerLimitBoundUnits=rad  LowerLimitStiffness=1e4  LowerLimitStiffnessUnits=N*m/deg  LowerLimitDamping=10  LowerLimitDampingUnits=N*m/(deg/s)  LowerLimitTransitionRegionWidth=0.1  LowerLimitTransitionRegionWidthUnits=deg  UpperLimitSpecify=on  UpperLimitBound=6.283185307179586  UpperLimitBoundUnits=rad  UpperLimitStiffness=1e4  UpperLimitStiffnessUnits=N*m/deg  UpperLimitDamping=10  UpperLimitDampingUnits=N*m/(deg/s)  UpperLimitTransitionRegionWidth=0.1  UpperLimitTransitionRegionWidthUnits=deg  TorqueActuationMode=ComputedTorque  MotionActuationMode=InputMotion  SensePosition=on  SenseVelocity=on  SenseAcceleration=off  SenseTorqueForce=off  SenseLowerLimitTorqueForce=off  SenseUpperLimitTorqueForce=off
  wrist_2_link : Subsystem
  wrist_3_flange : sm_lib/Joints/Weld Joint  JointMode=Normal  CompositeWrenchDir=FollowerOnBase  CompositeWrenchFrame=BaseFrame  SenseConstraintForce=off  SenseConstraintTorque=off  SenseTotalForce=off  SenseTotalTorque=off
  wrist_3_joint : sm_lib/Joints/Revolute Joint  JointMode=Normal  CompositeWrenchDir=FollowerOnBase  CompositeWrenchFrame=BaseFrame  SenseConstraintForce=off  SenseConstraintTorque=off  SenseTotalForce=off  SenseTotalTorque=off  PositionTargetSpecify=on  PositionTargetPriority=High  PositionTargetValue=initial_positions_rad(7)  PositionTargetValueUnits=rad  VelocityTargetSpecify=off  VelocityTargetPriority=High  VelocityTargetValue=0  VelocityTargetValueUnits=deg/s  EquilibriumPosition=0  EquilibriumPositionUnits=deg  SpringStiffness=0  SpringStiffnessUnits=N*m/deg  DampingCoefficient=0  DampingCoefficientUnits=kg*m^2/(rad*s)  LowerLimitSpecify=on  LowerLimitBound=-6.283185307179586  LowerLimitBoundUnits=rad  LowerLimitStiffness=1e4  LowerLimitStiffnessUnits=N*m/deg  LowerLimitDamping=10  LowerLimitDampingUnits=N*m/(deg/s)  LowerLimitTransitionRegionWidth=0.1  LowerLimitTransitionRegionWidthUnits=deg  UpperLimitSpecify=on  UpperLimitBound=6.283185307179586  UpperLimitBoundUnits=rad  UpperLimitStiffness=1e4  UpperLimitStiffnessUnits=N*m/deg  UpperLimitDamping=10  UpperLimitDampingUnits=N*m/(deg/s)  UpperLimitTransitionRegionWidth=0.1  UpperLimitTransitionRegionWidthUnits=deg  TorqueActuationMode=ComputedTorque  MotionActuationMode=InputMotion  SensePosition=on  SenseVelocity=on  SenseAcceleration=off  SenseTorqueForce=off  SenseLowerLimitTorqueForce=off  SenseUpperLimitTorqueForce=off
  wrist_3_link : Subsystem
  wrist_3_link_ft_frame : sm_lib/Joints/Weld Joint  JointMode=Normal  CompositeWrenchDir=FollowerOnBase  CompositeWrenchFrame=BaseFrame  SenseConstraintForce=off  SenseConstraintTorque=off  SenseTotalForce=off  SenseTotalTorque=off
  wires:
  Demux/1 -> XY Graph1/1, Gain/1
  Demux/2 -> XY Graph1/2, Gain1/1
  From Workspace3/1 -> MATLAB Function7/3(waypoints), Demux/1  "r3"
  MATLAB Function/1(dx_m) -> Integrator/1
  MATLAB Function1/1(dx_m) -> Integrator2/1
  Integrator2/1 -> Sum2/1, MATLAB Function1/1(x_m)
  MATLAB Function3/1(dx_m) -> Integrator3/1
  Integrator3/1 -> Sum4/1, MATLAB Function3/1(x_m)
  MATLAB Function4/1(dx) -> Integrator4/1
  Mux1/1 -> Sum1/1
  Sum1/1 -> Scope3/1, Selector4/1, Selector5/1, Selector9/1
  [r2] -> MATLAB Function1/2(r)
  Sum3/1 -> Scope4/1, MATLAB Function4/3(tau)
  Mux2/1 -> Sum3/2, Scope9/1
  Subsystem/1(tau_x) -> Mux2/1
  Integrator/1 -> Sum/1, MATLAB Function/1(x_m)
  Mux3/1 -> Sum/2
  [r1] -> MATLAB Function/2(r)
  Demux1/1 -> Mux3/1, MATLAB Function/3(theta_EQ)
  Sum/1 -> Mux1/1, Scope/1
  Demux1/2 -> Mux4/1, MATLAB Function1/3(theta_EQ)
  Mux4/1 -> Sum2/2
  Sum2/1 -> Scope11/1, Mux1/2
  Mux5/1 -> Sum4/2
  Sum4/1 -> Mux1/3
  EQ generator1/2(tau_EQ) -> Scope5/1, Sum3/1
  Constant1/1 -> Mux5/1, MATLAB Function3/2(r), [r3]  "r3"
  Selector3/1 -> Subsystem/2(frontal_x)  "frontal_x"
  Selector9/1 -> Subsystem/1(frontal_err)  "frontal_err"
  [r1] -> Subsystem/3(r1)
  [r2] -> Subsystem1/3(r2)
  [r3] -> Subsystem2/3(r3)
  Subsystem2/1(tau_z) -> Mux2/3
  Selector2/1 -> Subsystem1/2(saggital_y)  "saggital_y"
  Selector1/1 -> Subsystem2/2(transverse_y)
  Selector5/1 -> Subsystem1/1(saggital_err)  "saggital_err"
  Selector4/1 -> Subsystem2/1(transverse_err)  "transverse_err"
  Demux2/3 -> Gain5/1
  Demux2/7 -> Gain4/1
  Gain4/1 -> XY Graph/1  "r2"
  Gain5/1 -> XY Graph/2  "r2"
  PS-Simulink Converter7/1 -> Mux6/6
  Selector11/1 -> Demux3/1
  Integrator4/1 -> MATLAB Function2/1(x), Demux4/1, Demux2/1, Scope2/1, Sum1/2, Selector1/1, Selector2/1, Selector3/1, MATLAB Function7/1(x), MATLAB Function4/1(x)  "x"
  Demux3/3 -> Simulink-PS Converter4/1
  PS-Simulink Converter6/1 -> Mux6/5
  PS-Simulink Converter14/1 -> Mux9/1
  Demux4/9 -> Simulink-PS Converter13/1
  Detect Rise Positive/1 -> Triggered Subsystem/Trigger
  Demux3/2 -> Simulink-PS Converter3/1
  PS-Simulink Converter4/1 -> Mux6/3
  PS-Simulink Converter9/1 -> Mux7/2
  MATLAB Function5/1(simscape_true_trajectory) -> Selector11/1, Selector10/1
  Demux3/1 -> Simulink-PS Converter2/1
  PS-Simulink Converter3/1 -> Mux6/2
  Demux4/3 -> Multiply1/1
  Multiply1/1 -> Simulink-PS Converter8/1
  Mux9/1 -> Scope13/1
  Demux4/5 -> Simulink-PS Converter11/1
  Triggered Subsystem/1(trigger_time) -> Scope15/1, MATLAB Function5/1(trigger)
  PS-Simulink Converter11/1 -> Mux7/4
  PS-Simulink Converter12/1 -> Mux7/5
  Demux3/4 -> Simulink-PS Converter5/1
  Demux4/7 -> Multiply/1
  Mux8/1 -> [wrench]
  PS-Simulink Converter/1 -> Mux6/1
  Demux3/5 -> Simulink-PS Converter6/1
  Multiply/1 -> Simulink-PS Converter/1
  PS-Simulink Converter2/1 -> Mux8/2, Scope7/1
  Mux6/1 -> To Workspace/1, [q]
  Clock2/1 -> Triggered Subsystem/1(In1)
  PS-Simulink Converter8/1 -> Mux7/1
  Demux3/6 -> Simulink-PS Converter7/1
  PS-Simulink Converter15/1 -> Mux9/2
  PS-Simulink Converter1/1 -> Mux8/1, Scope6/1
  MATLAB Function2/1(cond) -> Detect Rise Positive/1
  Mux7/1 -> [q_dot]
  PS-Simulink Converter10/1 -> Mux7/3
  Selector10/1 -> Simulink-PS Converter1/1
  PS-Simulink Converter5/1 -> Mux6/4
  Demux4/1 -> Simulink-PS Converter10/1
  PS-Simulink Converter13/1 -> Mux7/6
  Subsystem1/1(tau_y) -> Mux2/2
  EQ generator1/1(theta_EQ) -> Demux1/1, Scope1/1
  [wrench] -> MATLAB Function4/2(wrench_ext), Scope8/1, Low-Pass Filter (Discrete or Continuous)/1
  Gain/1 -> Mux/2, [r2]
  Gain1/1 -> Mux/1, [r1]
  MATLAB Function7/1(phi_dot_c) -> EQ generator1/2(phi_dot_c)
  Clock/1 -> MATLAB Function7/2(simtime)
  Low-Pass Filter (Discrete or Continuous)/1 -> Demux5/1
  Mux10/1 -> EQ generator1/1(external_wrench)
  Demux5/1 -> Mux10/1
  Demux5/3 -> Mux10/3
  Demux5/5 -> Mux10/5
  connections:
  World/RConn1 -- Solver Configuration/RConn1 -- MechanismConfiguration/RConn1 -- world/LConn1
  PS Gain1/LConn1 -- PS Gain2/LConn1 -- PS Gain/LConn1 -- robotiq_85_left_knuckle_joint/RConn2
  robotiq_85_right_finger_tip_joint/LConn2 -- robotiq_85_left_inner_knuckle_joint/LConn2 -- robotiq_85_left_knuckle_joint/LConn2 -- Simulink-PS Converter1/RConn1
  wrist_1_joint/RConn1 -- wrist_1_link/LConn1
  robotiq_85_left_inner_knuckle_joint/RConn1 -- robotiq_85_left_inner_knuckle_link/LConn1
  PS-Simulink Converter2/LConn1 -- Gimbal Joint/RConn2
  wrist_2_joint/RConn3 -- PS-Simulink Converter12/LConn1
  forearm_link/RConn1 -- wrist_1_joint/LConn1
  robotiq_85_base_joint/RConn1 -- robotiq_85_base_link/LConn1
  wrist_1_link/RConn1 -- wrist_2_joint/LConn1
  base_link/RConn2 -- base_link_base_fixed_joint/LConn1
  PS-Simulink Converter1/LConn1 -- Cartesian Joint/RConn2
  wrist_2_joint/RConn2 -- PS-Simulink Converter6/LConn1
  shoulder_link/RConn1 -- shoulder_lift_joint/LConn1
  robotiq_85_right_finger_link/RConn1 -- robotiq_85_right_finger_tip_joint/LConn1
  PS-Simulink Converter14/LConn1 -- base_joint/RConn2
  wrist_3_link_ft_frame/RConn1 -- ft_frame/LConn1
  robotiq_85_base_link/RConn4 -- robotiq_85_left_inner_knuckle_joint/LConn1
  wrist_3_joint/RConn1 -- wrist_3_link/LConn1
  base_link/RConn1 -- base_link_base_link_inertia/LConn1
  robotiq_85_right_inner_knuckle_joint/RConn1 -- robotiq_85_right_inner_knuckle_link/LConn1
  upper_arm_link/RConn1 -- elbow_joint/LConn1
  Simulink-PS Converter5/RConn1 -- wrist_1_joint/LConn2
  PS-Simulink Converter4/LConn1 -- elbow_joint/RConn2
  base_joint/RConn1 -- base_link/LConn1
  Simulink-PS Converter13/RConn1 -- Gimbal Joint/LConn4
  robotiq_85_left_finger_joint/RConn1 -- robotiq_85_left_finger_link/LConn1
  Simulink-PS Converter3/RConn1 -- shoulder_lift_joint/LConn2
  shoulder_pan_joint/RConn3 -- PS-Simulink Converter8/LConn1
  ground_plane/LConn1 -- ground_plane_joint/RConn1
  ground_plane/RConn6 -- wrist_2_link/LConn2
  wrist_3_link/RConn2 -- wrist_3_flange/LConn1
  ground_plane/RConn3 -- upper_arm_link/LConn2
  ground_plane/RConn2 -- shoulder_link/LConn2
  wrist_1_joint/RConn2 -- PS-Simulink Converter5/LConn1
  robotiq_85_left_knuckle_joint/RConn1 -- robotiq_85_left_knuckle_link/LConn1
  wrist_2_link/RConn1 -- wrist_3_joint/LConn1
  robotiq_85_right_knuckle_link/RConn1 -- robotiq_85_right_finger_joint/LConn1
  robotiq_85_base_link/RConn3 -- robotiq_85_left_knuckle_joint/LConn1
  Simulink-PS Converter11/RConn1 -- Gimbal Joint/LConn3
  base_link_base_link_inertia/RConn1 -- base_link_inertia/LConn1
  ground_plane/RConn4 -- forearm_link/LConn2
  base_joint/LConn1 -- Transform/RConn1
  world/RConn2 -- Cartesian Joint/LConn1
  wrist_1_joint/RConn3 -- PS-Simulink Converter11/LConn1
  wrist_3_joint/RConn2 -- PS-Simulink Converter7/LConn1
  shoulder_pan_joint/RConn1 -- shoulder_link/LConn1
  robotiq_85_left_finger_link/RConn1 -- robotiq_85_left_finger_tip_joint/LConn1
  Cartesian Joint/RConn1 -- Gimbal Joint/LConn1
  robotiq_85_right_finger_joint/RConn1 -- robotiq_85_right_finger_link/LConn1
  robotiq_85_base_link/RConn2 -- robotiq_85_right_inner_knuckle_joint/LConn1
  PS Gain/RConn1 -- robotiq_85_right_inner_knuckle_joint/LConn2
  PS Gain1/RConn1 -- robotiq_85_right_knuckle_joint/LConn2
  elbow_joint/RConn1 -- forearm_link/LConn1
  flange/RConn2 -- flange_tool0/LConn1
  flange_tool0/RConn1 -- tool0/LConn1
  Simulink-PS Converter4/RConn1 -- elbow_joint/LConn2
  PS-Simulink Converter15/LConn1 -- base_joint/RConn3
  elbow_joint/RConn3 -- PS-Simulink Converter10/LConn1
  PS-Simulink Converter/LConn1 -- shoulder_pan_joint/RConn2
  Simulink-PS Converter8/RConn1 -- Cartesian Joint/LConn3
  shoulder_lift_joint/RConn1 -- upper_arm_link/LConn1
  shoulder_lift_joint/RConn3 -- PS-Simulink Converter9/LConn1
  PS Gain2/RConn1 -- robotiq_85_left_finger_tip_joint/LConn2
  wrist_3_joint/RConn3 -- PS-Simulink Converter13/LConn1
  robotiq_85_right_knuckle_joint/RConn1 -- robotiq_85_right_knuckle_link/LConn1
  Simulink-PS Converter2/RConn1 -- shoulder_pan_joint/LConn2
  robotiq_85_base_link/RConn1 -- robotiq_85_right_knuckle_joint/LConn1
  robotiq_85_right_finger_tip_joint/RConn1 -- robotiq_85_right_finger_tip_link/LConn1
  robotiq_85_left_finger_tip_joint/RConn1 -- robotiq_85_left_finger_tip_link/LConn1
  Simulink-PS Converter7/RConn1 -- wrist_3_joint/LConn2
  wrist_2_joint/RConn1 -- wrist_2_link/LConn1
  base_link_inertia/RConn1 -- shoulder_pan_joint/LConn1
  Simulink-PS Converter6/RConn1 -- wrist_2_joint/LConn2
  base_link_base_fixed_joint/RConn1 -- base/LConn1
  robotiq_85_left_knuckle_link/RConn1 -- robotiq_85_left_finger_joint/LConn1
  wrist_3_link/RConn1 -- wrist_3_link_ft_frame/LConn1
  shoulder_lift_joint/RConn2 -- PS-Simulink Converter3/LConn1
  world/RConn1 -- ground_plane_joint/LConn1
  wrist_3_flange/RConn1 -- flange/LConn1
  Simulink-PS Converter10/RConn1 -- Gimbal Joint/LConn2
  ground_plane/RConn5 -- wrist_1_link/LConn2
  flange/RConn1 -- robotiq_85_base_joint/LConn1
  Simulink-PS Converter/RConn1 -- Cartesian Joint/LConn2
  Transform/LConn1 -- Gimbal Joint/RConn1
  ground_plane/RConn7 -- wrist_3_link/LConn2
  ground_plane/RConn1 -- base_link_inertia/LConn2
